simulink model "mainEthan"  (R2023b)
settings: Solver=ode113  StartTime=tstart  StopTime=tend  RelTol=relTol  AbsTol=absTol
values from neighbouring files (symbols this model uses):
  DCM_initial = targetDCM([26321453.5527815,	-132781955.130633,	-57571626.5531097]', R_princ)    [EulerEquations.m]    (also in main_script.m)
  inertia_p = [85.075, 0, 0; 0, 85.075, 0; 0, 0, 120.2515]    [omega_dot.m]
  omega_init = [0; 0; 0.01]    [EulerEquations.m]    (also in main_script.m)
  state_ECI_init = [R_PQW_IJK*state_PQW_init(1:3)';R_PQW_IJK*state_PQW_init(4:6)']    [OrbitPropagation.m]
  theta = UT1_to_theta(UT1)    [EulerEquations.m]    (also in UT1_to_theta.m = rotz(-GMST*180/pi); main_script.m)
  tstart = 0    [EulerEquations.m]    (also in main_script.m)
  UT1 = [1,25,2004,00]    [EulerEquations.m]    (also in main_script.m)
undefined symbols (not defined in the file or in its folder): A, A_star, I_w, max_dipole, max_wheel_om, max_wheel_torque, omega_w_init, R_princ
libraries: simulink x4, dspmathops x3, aerolibatmos2 x1, matrix_library x1
(part 2 of 2)

== matlab function mainEthan/Environment Petrubations/Compute Air Density/MATLAB Function ==
  data: r_ECI input; geodetic output
function geodetic = fcn(r_ECI)
    rE = 6378;
    h = norm(r_ECI) - rE;
    lat = atan2(r_ECI(3), sqrt(r_ECI(1)^2 + r_ECI(2)^2));
    long = atan2(r_ECI(2), r_ECI(1));
    geodetic = [lat, long, h*1000];
end

== matlab function mainEthan/Attitude Estimation/Quaternions/Initial Quaternions ==
  data: C input; quaternions_init output
%% Quaternions
function quaternions_init = inital_quaternions(C)
    beta_4sq = (0.25*(1+trace(C)));
    beta_1sq = (0.25*(1+2*C(1,1)- trace(C)));
    beta_2sq = (0.25*(1+2*C(2,2)- trace(C)));
    beta_3sq = (0.25*(1+2*C(3,3)- trace(C)));
    
    [maximum, max_ind] = max([beta_1sq, beta_2sq, beta_3sq, beta_4sq]);
    
    switch max_ind
        case 1
            beta_1 = sqrt(beta_1sq);
            beta_4 = (C(2,3) - C(3,2))/(4*beta_1);
            beta_3 = (C(3,1) + C(1,3))/(4*beta_1);
            beta_2 = (C(1,2) + C(2,1))/(4*beta_1);
        case 2
            beta_2 = sqrt(beta_2sq);
            beta_4 = (C(3,1) - C(1,3))/(4*beta_2);
            beta_3 = (C(2,3) + C(3,2))/(4*beta_2);
            beta_1 = (C(1,2) + C(2,1))/(4*beta_2);
        case 3
            beta_3 = sqrt(beta_3sq);
            beta_4 = (C(1,2) - C(2,1))/(4*beta_3);
            beta_2 = (C(2,3) + C(3,2))/(4*beta_3);
            beta_1 = (C(3,1) + C(1,3))/(4*beta_3);
           
        otherwise
            beta_4 = sqrt(beta_4sq);
            beta_3 = (C(1,2) - C(2,1))/(4*beta_4);
            beta_2 = (C(3,1) - C(1,3))/(4*beta_4);
            beta_1 = (C(2,3) - C(3,2))/(4*beta_4);   
    end
    
    quaternions_init = [beta_1; beta_2; beta_3; beta_4];
    quaternions_init =  quaternions_init/ norm(quaternions_init); %normalize
end

== matlab function mainEthan/Attitude Estimation/Quaternions/Kinematic Equations Quaternions  ==
  data: omega input; quaternion input; quat_dot output
%% Kinematic Equation of motion quaternions
function quat_dot = quaternions_dot(omega, quaternion)
    Sigma = [0, omega(3), -omega(2), omega(1);
            -omega(3), 0, omega(1), omega(2);
            omega(2), -omega(1), 0, omega(3);
            -omega(1), -omega(2), -omega(3), 0];
    quat_dot = 0.5 * Sigma * quaternion;
end

== matlab function mainEthan/Spacecraft Subsystem/Measurement Generation ==
  data: sunsensor output; Rot input; sunsensor_gt input; rand_sun input; magnetometer_gt input; rand_magnet input; startracker_1_gt input; startracker_2_gt input; rand_star input; magnetometer output; startracker_1 output; startracker_2 output
%% return sensor measurements from ground truth

function [sunsensor, magnetometer, startracker_1, startracker_2] = measurement_generation(Rot, sunsensor_gt, rand_sun, magnetometer_gt, rand_magnet, startracker_1_gt, startracker_2_gt, rand_star)
    magnetometer = Rot * magnetometer_gt;
    magnetometer = [magnetometer(1)*(1+rand_magnet(1)); magnetometer(2)*(1+rand_magnet(2)); magnetometer(3)*(1+rand_magnet(3))];
    sunsensor = Rot*sunsensor_gt;
    sunsensor = rotationMatrix_z(rand_sun(1))*rotationMatrix(cross([sunsensor(1:2);0], [0; 0;1]), rand_sun(2))*sunsensor;
    startracker_1 = Rot * startracker_1_gt;
    startracker_2 = Rot * startracker_2_gt;
    for i = 1:length(startracker_1(1,:))
       startracker_1(:, i) = rotationMatrix_z(rand_star(1, i))*rotationMatrix(cross([startracker_1(1:2, i);0], [0; 0;1]), rand_star(2, i))*startracker_1(:, i);
       startracker_2(:, i) = rotationMatrix_z(rand_star(3, i))*rotationMatrix(cross([startracker_2(1:2, i);0], [0; 0;1]), rand_star(4, i))*startracker_2(:, i);
    end


end
function R = rotationMatrix(axis, angle)
    axis = axis ./ norm(axis);
    x = axis(1);
    y = axis(2);
    z = axis(3);
    c = cosd(angle);
    s = sind(angle);
    t = 1 - c;

    R = [t*x*x + c,    t*x*y - s*z,  t*x*z + s*y;
         t*x*y + s*z,  t*y*y + c,    t*y*z - s*x;
         t*x*z - s*y,  t*y*z + s*x,  t*z*z + c];
end

function R_z = rotationMatrix_z(angle)
    c = cosd(angle);
    s = sind(angle);
    
    % Construct the rotation matrix around the z-axis
    R_z = [c, -s, 0;
         s,  c, 0;
         0,  0, 1];
end

== matlab function mainEthan/Spacecraft Subsystem/Reference Truth ==
  data: sunsensor output; magnetometer output; Rot input; magnetic_field input; r_sun input; startracker_1 output; startracker_2 output
%% return ground truth in ECI
function [sunsensor,  magnetometer, startracker_1, startracker_2] = reference_truth(Rot, magnetic_field, r_sun)
    magnetometer = Rot'*magnetic_field; 
    sunsensor = r_sun(1:3)./norm(r_sun(1:3)); %already in ECI
    startracker_1 = zeros(3, 15);
    startracker_2 = zeros(3, 15);
    for i = 1:length(startracker_1(1,:))
        RA1 = 75 + i;
        declination1 = 35 + i;
        startracker_1(:, i) = Rot'*[cosd(RA1)*cosd(declination1); sind(RA1)*cosd(declination1); sind(declination1)]; %target for body z-axis
        RA2 = 250 + i;
        declination2 = 12 + i;
        startracker_2(:, i) = Rot'*[cosd(RA2)*cosd(declination2); sind(RA2)*cosd(declination2); sind(declination2)]; %target for body z-axis
    end
end

== matlab function mainEthan/Spacecraft Subsystem/Hardware Measurements ==
  data: R_princ input; DCM input; sun_sensor_noise input; B input; mag_noise input; sunsensor output; r_sun input; magnetometer output
%% return ground truth in ECI
function [sunsensor, magnetometer]  = hardware_measurements(R_princ, DCM, sun_sensor_noise, B, mag_noise, r_sun)
    sun_sensor_normal = R_princ*[0,0,1]'; % Sensor Direction in Principal
    r_sun = DCM*r_sun; % Sun in Principal 
    r_sun_unit = r_sun/norm(r_sun); % Sun Unit in Principal
    
    % Sun Sensor, 4 quadrant voltage plates 
    % % Angles of Sun Vector 
    % theta_x = atan2(r_sun_unit(1),r_sun_unit(3));
    % theta_y = atan2(r_sun_unit(2),r_sun_unit(3));
    % 
    % % Sun Sensor Hardware 
    % V_max = 5; % Output 0 to 5 Volts
    % 
    % % Voltage on Each Quadrant Plus Noise 
    % V_A = V_max*max(0,r_sun_unit(3) + r_sun_unit(1) + r_sun_unit(2)) + sun_sensor_noise(1);
    % V_B = V_max*max(0,r_sun_unit(3) + r_sun_unit(1) - r_sun_unit(2)) + sun_sensor_noise(2);
    % V_C = V_max*max(0,r_sun_unit(3) - r_sun_unit(1) + r_sun_unit(2)) + sun_sensor_noise(3);
    % V_D = V_max*max(0,r_sun_unit(3) - r_sun_unit(1) - r_sun_unit(2)) + sun_sensor_noise(4);
    % 
    % % if V_A < 0
    % %     V_A = 0;
    % % elseif V_A > 5;
    % %     V_A = 5;
    % % else
    % %     V_A = V_A; 
    % % end
    % % 
    % % if V_B < 0
    % %     V_B = 0;
    % % elseif V_B > 5;
    % %     V_B = 5;
    % % else
    % %     V_B = V_B; 
    % % end
    % % 
    % % if V_C < 0
    % %     V_C = 0;
    % % elseif V_C > 5;
    % %     V_C = 5;
    % % else
    % %     V_C = V_C; 
    % % end
    % % 
    % % if V_D < 0
    % %     V_D = 0;
    % % elseif V_D > 5;
    % %     V_D = 5;
    % % else
    % %     V_D = V_D; 
    % % end
    % 
    % % See or not 
    % theta_StoNormal = acos(dot(sun_sensor_normal_unit, r_sun_unit)); % Angle Between
    % if theta_StoNormal >= 0 && theta_StoNormal <= pi/2
    %     % Get sun unit vector from voltages
    %     V_tot = V_A + V_B + V_C + V_D;
    %     V_A_n = V_A/V_tot;
    %     V_B_n = V_B/V_tot;
    %     V_C_n = V_C/V_tot;
    %     V_D_n = V_D/V_tot;
    % 
    %     V_x = (V_A_n + V_B_n) - (V_C_n + V_D_n);
    %     V_y = (V_A_n + V_C_n) - (V_B_n + V_D_n);
    %     sumSquares = V_x^2 + V_y^2;
    %     if sumSquares > 1
    %         % Clamp the sum of squares to 1 if it exceeds
    %         scale = 1 / sqrt(sumSquares);
    %         V_x = V_x * scale;
    %         V_y = V_y * scale;
    %         V_z = 0;  % If the sum of squares exceeds 1, set I_z to 0 (horizon)
    %     else
    %         % Calculate the z component
    %         V_z = sqrt(1 - sumSquares);
    %     end
    % 
    %     % Reconstruct the sun vector 
    %     sunsensor = [V_x,V_y,V_z]';
    % else
    %     sunsensor = [0,0,0]';
    % end

    % Sun Sensor, simple model 
    V_max = 5; % Voltage when r_sun perpendicular
    theta_StoNormal = acos(dot(sun_sensor_normal, r_sun_unit)); % Angle Between
    V_noisy = V_max*cos(theta_StoNormal) + sun_sensor_noise;

    if V_noisy > 5
        V_noisy = 5;
    elseif V_noisy < -5
        V_noisy = -5;
    else
        V_noisy = V_noisy;
    end

    theta_new = acos(V_noisy/V_max);
    theta_noise = theta_new - theta_StoNormal;
    sunsensor = rotationMatrix_z(theta_noise)*rotationMatrix(cross([r_sun_unit(1:2);0], [0; 0;1]), theta_noise)*r_sun_unit;
    
    % Magnetometer, B in ECI
    B = DCM*B; % B in Principal;
    B = (R_princ')*B; % B in Body;
    S = 100*1000; % Sensitivity in V/T
    bias = 0.025; % Volt Bias

    % Calculate Voltage and Apply Noise and Bias
    V_x_mag = S*B(1) + bias + mag_noise(1);
    V_y_mag = S*B(2) + bias + mag_noise(2);
    V_z_mag = S*B(3) + bias + mag_noise(3);
    
    % Go back to magnetic field vector components
    magnetometer = [(V_x_mag - bias)/S, (V_y_mag - bias)/S, (V_z_mag - bias)/S]';
    magnetometer = (R_princ)*magnetometer; % Back to Principal
    magnetometer = (DCM')*magnetometer;
end
function R = rotationMatrix(axis, angle)
    axis = axis ./ norm(axis);
    x = axis(1);
    y = axis(2);
    z = axis(3);
    c = cos(angle);
    s = sin(angle);
    t = 1 - c;

    R = [t*x*x + c,    t*x*y - s*z,  t*x*z + s*y;
         t*x*y + s*z,  t*y*y + c,    t*y*z - s*x;
         t*x*z - s*y,  t*y*z + s*x,  t*z*z + c];
end

function R_z = rotationMatrix_z(angle)
    c = cos(angle);
    s = sin(angle);
    
    % Construct the rotation matrix around the z-axis
    R_z = [c, -s, 0;
         s,  c, 0;
         0,  0, 1];
end

== matlab function mainEthan/Close Loop ==
  data: x_est input; omega output; DCM output
function [omega, DCM] = state2om_DCM(x_est)
    quaternions = x_est(4:end);
    q1 = quaternions(1);
    q2 = quaternions(2);
    q3 = quaternions(3);
    q4 = quaternions(4);
    omega = x_est(1:3);
    DCM = (q4^2 - norm(quaternions(1:3))^2) * eye(3,3) + 2*quaternions(1:3)*quaternions(1:3)' -2*q4*[0, -q3, q2; q3, 0, -q1; -q2, q1, 0];
 
end

== matlab function mainEthan/Attitude/Quaternions/Kinematic Equations Quaternions  ==
  data: omega input; quaternion input; quat_dot output
%% Kinematic Equation of motion quaternions
function quat_dot = quaternions_dot(omega, quaternion)
    Sigma = [0, omega(3), -omega(2), omega(1);
            -omega(3), 0, omega(1), omega(2);
            omega(2), -omega(1), 0, omega(3);
            -omega(1), -omega(2), -omega(3), 0];
    quat_dot = 0.5 * Sigma * quaternion;
end

== matlab function mainEthan/Euler Equations/Euler Equations1 ==
  data: inertia_p input; M input; M_c input; omegadot output; omega input
%% return omega_dot (zero torque)
function omegadot  = omega_dot(inertia_p, M, M_c, omega)
    %Euler eqns in principal axes
    omegadot = [ 1/inertia_p(1,1) * (M(1) + M_c(1) - (inertia_p(3,3) - inertia_p(2,2)) * omega(2)*omega(3));
                 1/inertia_p(2,2) * (M(2) + M_c(2) - (inertia_p(1,1) - inertia_p(3,3)) * omega(3)*omega(1));
                 1/inertia_p(3,3) * (M(3) + M_c(3) - (inertia_p(2,2) - inertia_p(1,1)) * omega(1)*omega(2))];
end

== matlab function mainEthan/Attitude/Quaternions/Initial Quaternions ==
  data: C input; quaternions_init output
%% Quaternions
function quaternions_init = inital_quaternions(C)
    beta_4sq = (0.25*(1+trace(C)));
    beta_1sq = (0.25*(1+2*C(1,1)- trace(C)));
    beta_2sq = (0.25*(1+2*C(2,2)- trace(C)));
    beta_3sq = (0.25*(1+2*C(3,3)- trace(C)));
    
    [maximum, max_ind] = max([beta_1sq, beta_2sq, beta_3sq, beta_4sq]);
    
    switch max_ind
        case 1
            beta_1 = sqrt(beta_1sq);
            beta_4 = (C(2,3) - C(3,2))/(4*beta_1);
            beta_3 = (C(3,1) + C(1,3))/(4*beta_1);
            beta_2 = (C(1,2) + C(2,1))/(4*beta_1);
        case 2
            beta_2 = sqrt(beta_2sq);
            beta_4 = (C(3,1) - C(1,3))/(4*beta_2);
            beta_3 = (C(2,3) + C(3,2))/(4*beta_2);
            beta_1 = (C(1,2) + C(2,1))/(4*beta_2);
        case 3
            beta_3 = sqrt(beta_3sq);
            beta_4 = (C(1,2) - C(2,1))/(4*beta_3);
            beta_2 = (C(2,3) + C(3,2))/(4*beta_3);
            beta_1 = (C(3,1) + C(1,3))/(4*beta_3);
           
        otherwise
            beta_4 = sqrt(beta_4sq);
            beta_3 = (C(1,2) - C(2,1))/(4*beta_4);
            beta_2 = (C(3,1) - C(1,3))/(4*beta_4);
            beta_1 = (C(2,3) - C(3,2))/(4*beta_4);   
    end
    
    quaternions_init = [beta_1; beta_2; beta_3; beta_4];
    quaternions_init =  quaternions_init/ norm(quaternions_init); %normalize
end

== matlab function mainEthan/Attitude/Euler Angles/Euler Equations Euler ==
  data: omega input; euler input; eulerdot output
%% Kinematic Equation of motion for euler angles [phi, theta, psi]
function eulerdot = euler_dot(omega, euler)
     % phi_dot = (omega(1)* sin(euler(3)) + omega(2)*cos(euler(3)))/sin(euler(2));
     % theta_dot = omega(1) * cos(euler(3)) - omega(2) * sin(euler(3));
     % psi_dot = omega(3) - (omega(1)* sin(euler(3)) + omega(2)*cos(euler(3))) * cot(euler(2));
     % eulerdot = [phi_dot, theta_dot, psi_dot];
     phi = euler(1);
     theta = euler(2);
     psi = euler(3);

     eulerdot = 1/sin(theta)*[-sin(phi)*cos(theta), -cos(phi)*cos(theta), sin(theta);
                            cos(phi)*sin(theta), -sin(phi)*sin(theta), 0;
                            sin(phi), cos(phi), 0] * omega;
end

== matlab function mainEthan/Attitude/Euler Angles/Initial Euler Angles ==
  data: C input; euler_init output
%% Euler Angles
function  euler_init = inital_euler(C)
    phi = atan2(C(1,3), C(2,3));
    theta = acos(C(3,3));
    psi = atan2(C(3,1), -C(3,2));
    euler_init = [phi; theta; psi];
end

== matlab function mainEthan/Attitude/Euler Angles/Principal -> Inertial (Euler) ==
  data: euler input; omega_inertial_euler output; omega input; inertia_p input; A input; I_w input; L_inertial_euler output; R output; omega_w input
%% Transform Omega in inertial frame using Euler Angles
function [omega_inertial_euler, L_inertial_euler, R ] = principal_to_inertial(euler, omega, inertia_p, A, I_w, omega_w)
    phi = euler(1);
    theta = euler(2);
    psi = euler(3);
    
    Rz = @(x)[cos(x), sin(x), 0;
              -sin(x), cos(x), 0;
              0, 0, 1];
    Rx =  @(x)[1, 0, 0;
              0, cos(x), sin(x),;
              0, -sin(x), cos(x)];


    %R = Rz(euler(1))*Rx(euler(2))*Rz(euler(3));

    R = [cos(phi)*cos(psi) - sin(phi)*cos(theta)*sin(psi), cos(phi)*sin(psi)+sin(phi)*cos(theta)*cos(psi), sin(phi)*sin(theta);
        -sin(phi)*cos(psi) - cos(phi)*cos(theta)*sin(psi), -sin(phi)*sin(psi)+cos(phi)*cos(theta)*cos(psi), cos(phi)*sin(theta);
        sin(theta)*sin(psi), -sin(theta)*cos(psi), cos(theta)];
    
    omega_inertial_euler = R' * omega;
    %inertia_inertial = R * inertia_p * R';
    %L_inertial_euler = inertia_inertial * omega_inertial_euler;
    L_inertial_euler = R' * inertia_p * omega + A*(I_w*omega_w);
end

== matlab function mainEthan/Attitude/Quaternions/Principal -> Inertial (Quat) ==
  data: quaternions input; omega_inertial_quat output; omega input; inertia_p input; L_inertial_quat output; R output; A input; I_w input; omega_w input
%% Transform Omega in inertial frame using Quaternions
function  [omega_inertial_quat, L_inertial_quat, R] = principal_to_inertial(quaternions, omega, inertia_p, A, I_w, omega_w)
    q4 = quaternions(4);
    q1 = quaternions(1);
    q2 = quaternions(2);
    q3 = quaternions(3);
    % R = [q0^2+q1^2-q2^2-q3^2, 2*q1*q2 + 2*q0*q3, 2*q1*q3 - 2*q0*q2;
    %      2*q1*q2 - 2*q0*q3, q0^2 - q1^2+q2^2 - q3^2, 2*q2*q3 + 2*q0*q1;
    %      2*q1*q3 + 2*q0*q2, 2*q2*q3 - 2*q0*q1, q0^2-q1^2-q2^2 + q3^2];
    R = (q4^2 - norm(quaternions(1:3))^2) * eye(3,3) + 2*quaternions(1:3)*quaternions(1:3)' -2*q4*[0, -q3, q2; q3, 0, -q1; -q2, q1, 0];
    omega_inertial_quat = R' * omega;
    L_inertial_quat = R' * inertia_p * omega + A*(I_w*omega_w);
end
